simulink model "experiment_data_recording"  (Simulink 8.3)
settings: Solver=FixedStepDiscrete  StartTime=0.0  StopTime=inf  FixedStep=Ts  RelTol=1e-3
InitFcn:
  | robotName = 'icub';
  | localName = 'record_my_experiment';
  | Ts = 0.01;
  | ROBOT_DOF = 25;
libraries: WBCLibrary x2, utility x1
settings Model: Creator=talha  LastModifiedBy=talha
settings DataIOCC: SignalLoggingSaveFormat=Dataset
settings DebuggingCC: UnderspecifiedInitializationDetection=Simplified  StateNameClashWarn=none
settings GRTTargetCC: CombineOutputUpdateFcns=on  GRTInterface=off

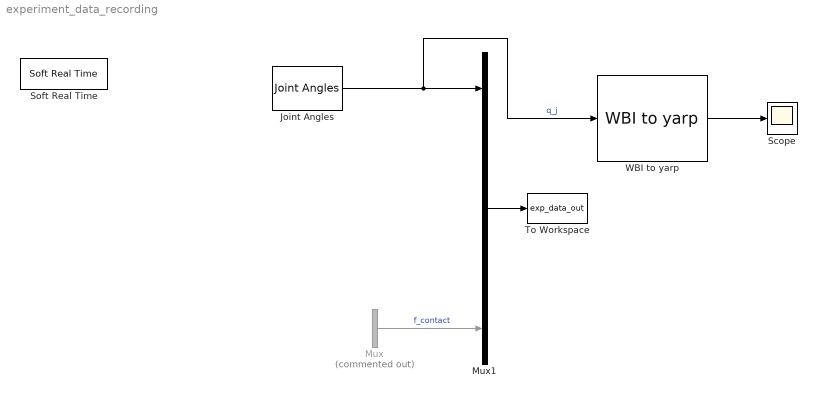
== system experiment_data_recording ==
  Joint Angles : WBCLibrary/wholeBodyStates/Joint Angles  robotName=robotName  localName=localName
  Mux : Mux  Commented=on  Inputs=2
  Mux1 : Mux
  Scope : Scope
      settings: YMin=-0.55  YMax=0.6
  Soft Real Time : utility/Soft Real Time  x=1
  To Workspace : ToWorkspace  VariableName=exp_data_out  SaveFormat=Timeseries  SampleTime=-1
  WBI to yarp : WBCLibrary/Utilities/WBI to yarp
  wires:
  ? -> Mux/2
  ? -> Mux/1
  Mux/1 -> Mux1/4  "f_contact"
  ? -> Mux1/2  "x_com"
  Joint Angles/1 -> WBI to yarp/1, Mux1/1  "q_j"
  Mux1/1 -> To Workspace/1
  WBI to yarp/3 -> Scope/1
